simulink model "SigProcess"  (R2022b)
settings: Solver=FixedStepDiscrete  StartTime=0.0  StopTime=10.0  FixedStep=0.001  RelTol=1e-3
undefined symbols (not defined in the file): cClCddAdc_D_u16ADNum, cClCddAdc_D_u8FilterType, cClCddAdc_D_u8RawValueNum, cTmAfCtrl_Te_s32ShttrPosnColdOnHp
libraries: simulink x132
(part 4 of 7)

== system SigProcess/SigProcessSub/Stp4_createSubModInfo/CLHB02001_AdFilter/AVG6 ==
  sigin : Inport
  Compare To Constant : simulink/Logic and Bit Operations/Compare To Constant  relop===  const=0  OutDataTypeStr=boolean
  Constant : Constant  Value=cClCddAdc_D_u8FilterType  OutDataTypeStr=uint8
  Constant1 : Constant  Value=cClCddAdc_D_u8RawValueNum  OutDataTypeStr=uint8
  Counter Limited : simulink/Sources/Counter Limited  uplimit=cClCddAdc_D_u8RawValueNum-1  tsamp=-1
  Data Store Memory : DataStoreMemory  DataStoreName=TempFlapFroLiFbRaw  ReadBeforeWriteMsg=warning  WriteAfterWriteMsg=warning  WriteAfterReadMsg=warning  ShowAdditionalParam=off  OutDataTypeStr=single  Dimensions=[1 20]
      settings: CopyFcn=set_param(gcbh,'ShowName','off');
  Data Store Read : DataStoreRead  DataStoreName=TempFlapFroLiFbRaw  IndexOptions=Index vector (dialog)  Indices=1  OutputSizes=1
  Data Store Write : DataStoreWrite  DataStoreName=TempFlapFroLiFbRaw  DataStoreElements=TempFlapFroLiFbRaw  EnableIndexing=on  IndexMode=Zero-based  IndexOptions=Index vector (port)  Indices=1  OutputSizes=1
  Data Type Conversion : DataTypeConversion  OutDataTypeStr=single  SaturateOnIntegerOverflow=off  RndMeth=Floor
  Gain1 : Gain  Gain=1/cClCddAdc_D_u8RawValueNum
  MATLAB Function : MATLAB Function  TreatAsAtomicUnit=on
  Multiport Switch : MultiPortSwitch  DataPortOrder=Zero-based contiguous  Inputs=5  DataPortForDefault=Additional data port  zeroidx=on  OutDataTypeStr=single  SaturateOnIntegerOverflow=off  InputSameDT=off
  Scope : Scope
  Sum of Elements1 : Sum  Inputs=+
  Switch : Switch  Criteria=u2 ~= 0  SaturateOnIntegerOverflow=off  InputSameDT=off
  Unit Delay : UnitDelay  SampleTime=-1  HasFrameUpgradeWarning=on
  sigAvg : Outport  OutDataTypeStr=single
  wires:
  Data Store Read/1 -> MATLAB Function/1(u), Sum of Elements1/1
  Sum of Elements1/1 -> Gain1/1
  Compare To Constant/1 -> Switch/2
  Switch/1 -> [sigAvgSimple], Unit Delay/1
  Gain1/1 -> Switch/1, [sigAvgQuick]
  Counter Limited/1 -> Compare To Constant/1, Data Store Write/2
  Data Type Conversion/1 -> [siginSingle], Data Store Write/1, Scope/1
  MATLAB Function/2(withoutEdge) -> [sigAvgSortWithoutEdge]
  Unit Delay/1 -> Switch/3
  MATLAB Function/1(mid) -> [sigAvgSortedMid]
  sigin/1 -> [sigin]
  [sigin] -> Data Type Conversion/1
  [sigin] -> Multiport Switch/7
  Constant/1 -> Multiport Switch/1
  [sigAvgSortedMid] -> Multiport Switch/3
  [sigAvgSortWithoutEdge] -> Multiport Switch/4
  [sigAvgSimple] -> Multiport Switch/5
  [sigAvgQuick] -> Multiport Switch/6
  [siginSingle] -> Multiport Switch/2
  Multiport Switch/1 -> [sigAvg]
  [sigAvg] -> sigAvg/1
  Constant1/1 -> MATLAB Function/2(num)

== system SigProcess/SigProcessSub/Stp4_createSubModInfo/CLHB02001_AdFilter/AVG7 ==
  sigin : Inport
  Compare To Constant : simulink/Logic and Bit Operations/Compare To Constant  relop===  const=0  OutDataTypeStr=boolean
  Constant : Constant  Value=cClCddAdc_D_u8FilterType  OutDataTypeStr=uint8
  Constant1 : Constant  Value=cClCddAdc_D_u8RawValueNum  OutDataTypeStr=uint8
  Counter Limited : simulink/Sources/Counter Limited  uplimit=cClCddAdc_D_u8RawValueNum-1  tsamp=-1
  Data Store Memory : DataStoreMemory  DataStoreName=TempFlapFroRIFbRaw  ReadBeforeWriteMsg=warning  WriteAfterWriteMsg=warning  WriteAfterReadMsg=warning  ShowAdditionalParam=off  OutDataTypeStr=single  Dimensions=[1 20]
      settings: CopyFcn=set_param(gcbh,'ShowName','off');
  Data Store Read : DataStoreRead  DataStoreName=TempFlapFroRIFbRaw  IndexOptions=Index vector (dialog)  Indices=1  OutputSizes=1
  Data Store Write : DataStoreWrite  DataStoreName=TempFlapFroRIFbRaw  DataStoreElements=TempFlapFroRIFbRaw  EnableIndexing=on  IndexMode=Zero-based  IndexOptions=Index vector (port)  Indices=1  OutputSizes=1
  Data Type Conversion : DataTypeConversion  OutDataTypeStr=single  SaturateOnIntegerOverflow=off  RndMeth=Floor
  Gain1 : Gain  Gain=1/cClCddAdc_D_u8RawValueNum
  MATLAB Function : MATLAB Function  TreatAsAtomicUnit=on
  Multiport Switch : MultiPortSwitch  DataPortOrder=Zero-based contiguous  Inputs=5  DataPortForDefault=Additional data port  zeroidx=on  OutDataTypeStr=single  SaturateOnIntegerOverflow=off  InputSameDT=off
  Scope : Scope
  Sum of Elements1 : Sum  Inputs=+
  Switch : Switch  Criteria=u2 ~= 0  SaturateOnIntegerOverflow=off  InputSameDT=off
  Unit Delay : UnitDelay  SampleTime=-1  HasFrameUpgradeWarning=on
  sigAvg : Outport  OutDataTypeStr=single
  wires:
  Constant1/1 -> MATLAB Function/2(num)
  [sigAvg] -> sigAvg/1
  Multiport Switch/1 -> [sigAvg]
  [siginSingle] -> Multiport Switch/2
  [sigAvgQuick] -> Multiport Switch/6
  [sigAvgSimple] -> Multiport Switch/5
  [sigAvgSortWithoutEdge] -> Multiport Switch/4
  [sigAvgSortedMid] -> Multiport Switch/3
  Constant/1 -> Multiport Switch/1
  [sigin] -> Multiport Switch/7
  [sigin] -> Data Type Conversion/1
  sigin/1 -> [sigin]
  MATLAB Function/1(mid) -> [sigAvgSortedMid]
  Unit Delay/1 -> Switch/3
  MATLAB Function/2(withoutEdge) -> [sigAvgSortWithoutEdge]
  Data Type Conversion/1 -> Scope/1, Data Store Write/1, [siginSingle]
  Counter Limited/1 -> Data Store Write/2, Compare To Constant/1
  Gain1/1 -> [sigAvgQuick], Switch/1
  Switch/1 -> Unit Delay/1, [sigAvgSimple]
  Compare To Constant/1 -> Switch/2
  Sum of Elements1/1 -> Gain1/1
  Data Store Read/1 -> Sum of Elements1/1, MATLAB Function/1(u)

== system SigProcess/SigProcessSub/Stp4_createSubModInfo/CLHB02001_AdFilter/AVG8 ==
  sigin : Inport
  Compare To Constant : simulink/Logic and Bit Operations/Compare To Constant  relop===  const=0  OutDataTypeStr=boolean
  Constant : Constant  Value=cClCddAdc_D_u8FilterType  OutDataTypeStr=uint8
  Constant1 : Constant  Value=cClCddAdc_D_u8RawValueNum  OutDataTypeStr=uint8
  Counter Limited : simulink/Sources/Counter Limited  uplimit=cClCddAdc_D_u8RawValueNum-1  tsamp=-1
  Data Store Memory : DataStoreMemory  DataStoreName=ModFlapFroRIFbRaw  ReadBeforeWriteMsg=warning  WriteAfterWriteMsg=warning  WriteAfterReadMsg=warning  ShowAdditionalParam=off  OutDataTypeStr=single  Dimensions=[1 20]
      settings: CopyFcn=set_param(gcbh,'ShowName','off');
  Data Store Read : DataStoreRead  DataStoreName=ModFlapFroRIFbRaw  IndexOptions=Index vector (dialog)  Indices=1  OutputSizes=1
  Data Store Write : DataStoreWrite  DataStoreName=ModFlapFroRIFbRaw  DataStoreElements=ModFlapFroRIFbRaw  EnableIndexing=on  IndexMode=Zero-based  IndexOptions=Index vector (port)  Indices=1  OutputSizes=1
  Data Type Conversion : DataTypeConversion  OutDataTypeStr=single  SaturateOnIntegerOverflow=off  RndMeth=Floor
  Gain1 : Gain  Gain=1/cClCddAdc_D_u8RawValueNum
  MATLAB Function : MATLAB Function  TreatAsAtomicUnit=on
  Multiport Switch : MultiPortSwitch  DataPortOrder=Zero-based contiguous  Inputs=5  DataPortForDefault=Additional data port  zeroidx=on  OutDataTypeStr=single  SaturateOnIntegerOverflow=off  InputSameDT=off
  Scope : Scope
  Sum of Elements1 : Sum  Inputs=+
  Switch : Switch  Criteria=u2 ~= 0  SaturateOnIntegerOverflow=off  InputSameDT=off
  Unit Delay : UnitDelay  SampleTime=-1  HasFrameUpgradeWarning=on
  sigAvg : Outport  OutDataTypeStr=single
  wires:
  Data Store Read/1 -> MATLAB Function/1(u), Sum of Elements1/1
  Sum of Elements1/1 -> Gain1/1
  Compare To Constant/1 -> Switch/2
  Switch/1 -> [sigAvgSimple], Unit Delay/1
  Gain1/1 -> Switch/1, [sigAvgQuick]
  Counter Limited/1 -> Compare To Constant/1, Data Store Write/2
  Data Type Conversion/1 -> [siginSingle], Data Store Write/1, Scope/1
  MATLAB Function/2(withoutEdge) -> [sigAvgSortWithoutEdge]
  Unit Delay/1 -> Switch/3
  MATLAB Function/1(mid) -> [sigAvgSortedMid]
  sigin/1 -> [sigin]
  [sigin] -> Data Type Conversion/1
  [sigin] -> Multiport Switch/7
  Constant/1 -> Multiport Switch/1
  [sigAvgSortedMid] -> Multiport Switch/3
  [sigAvgSortWithoutEdge] -> Multiport Switch/4
  [sigAvgSimple] -> Multiport Switch/5
  [sigAvgQuick] -> Multiport Switch/6
  [siginSingle] -> Multiport Switch/2
  Multiport Switch/1 -> [sigAvg]
  [sigAvg] -> sigAvg/1
  Constant1/1 -> MATLAB Function/2(num)

== system SigProcess/SigProcessSub/Stp4_createSubModInfo/CLHB02001_AdFilter/AVG9 ==
  sigin : Inport
  Compare To Constant : simulink/Logic and Bit Operations/Compare To Constant  relop===  const=0  OutDataTypeStr=boolean
  Constant : Constant  Value=cClCddAdc_D_u8FilterType  OutDataTypeStr=uint8
  Constant1 : Constant  Value=cClCddAdc_D_u8RawValueNum  OutDataTypeStr=uint8
  Counter Limited : simulink/Sources/Counter Limited  uplimit=cClCddAdc_D_u8RawValueNum-1  tsamp=-1
  Data Store Memory : DataStoreMemory  DataStoreName=AqsPinRaw  ReadBeforeWriteMsg=warning  WriteAfterWriteMsg=warning  WriteAfterReadMsg=warning  ShowAdditionalParam=off  OutDataTypeStr=single  Dimensions=[1 20]
      settings: CopyFcn=set_param(gcbh,'ShowName','off');
  Data Store Read : DataStoreRead  DataStoreName=AqsPinRaw  IndexOptions=Index vector (dialog)  Indices=1  OutputSizes=1
  Data Store Write : DataStoreWrite  DataStoreName=AqsPinRaw  DataStoreElements=AqsPinRaw  EnableIndexing=on  IndexMode=Zero-based  IndexOptions=Index vector (port)  Indices=1  OutputSizes=1
  Data Type Conversion : DataTypeConversion  OutDataTypeStr=single  SaturateOnIntegerOverflow=off  RndMeth=Floor
  Gain1 : Gain  Gain=1/cClCddAdc_D_u8RawValueNum
  MATLAB Function : MATLAB Function  TreatAsAtomicUnit=on
  Multiport Switch : MultiPortSwitch  DataPortOrder=Zero-based contiguous  Inputs=5  DataPortForDefault=Additional data port  zeroidx=on  OutDataTypeStr=single  SaturateOnIntegerOverflow=off  InputSameDT=off
  Scope : Scope
  Sum of Elements1 : Sum  Inputs=+
  Switch : Switch  Criteria=u2 ~= 0  SaturateOnIntegerOverflow=off  InputSameDT=off
  Unit Delay : UnitDelay  SampleTime=-1  HasFrameUpgradeWarning=on
  sigAvg : Outport  OutDataTypeStr=single
  wires:
  Constant1/1 -> MATLAB Function/2(num)
  [sigAvg] -> sigAvg/1
  Multiport Switch/1 -> [sigAvg]
  [siginSingle] -> Multiport Switch/2
  [sigAvgQuick] -> Multiport Switch/6
  [sigAvgSimple] -> Multiport Switch/5
  [sigAvgSortWithoutEdge] -> Multiport Switch/4
  [sigAvgSortedMid] -> Multiport Switch/3
  Constant/1 -> Multiport Switch/1
  [sigin] -> Multiport Switch/7
  [sigin] -> Data Type Conversion/1
  sigin/1 -> [sigin]
  MATLAB Function/1(mid) -> [sigAvgSortedMid]
  Unit Delay/1 -> Switch/3
  MATLAB Function/2(withoutEdge) -> [sigAvgSortWithoutEdge]
  Data Type Conversion/1 -> Scope/1, Data Store Write/1, [siginSingle]
  Counter Limited/1 -> Data Store Write/2, Compare To Constant/1
  Gain1/1 -> [sigAvgQuick], Switch/1
  Switch/1 -> Unit Delay/1, [sigAvgSimple]
  Compare To Constant/1 -> Switch/2
  Sum of Elements1/1 -> Gain1/1
  Data Store Read/1 -> Sum of Elements1/1, MATLAB Function/1(u)

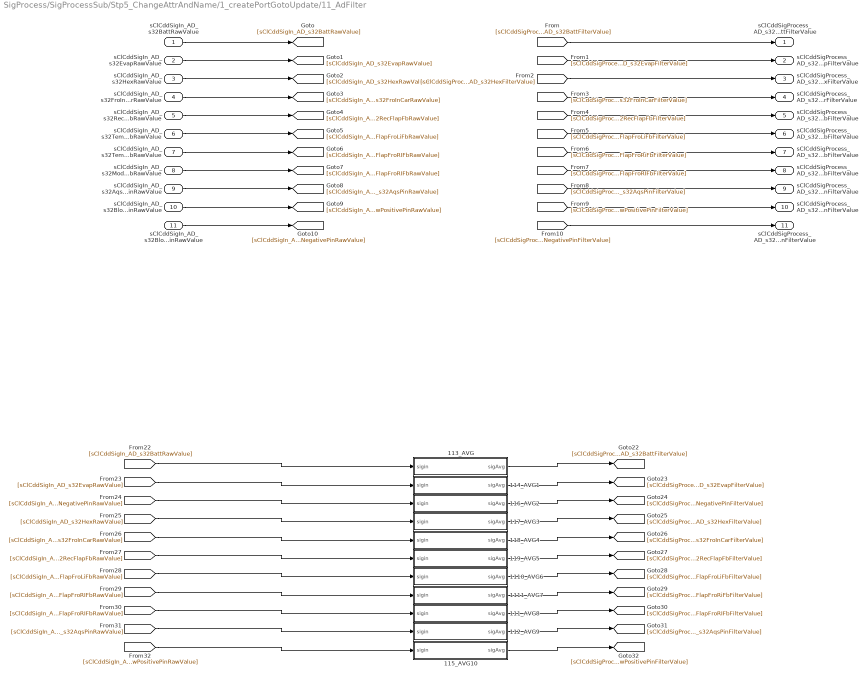
== system SigProcess/SigProcessSub/Stp5_ChangeAttrAndName/1_createPortGotoUpdate/11_AdFilter ==
  sClCddSigIn_AD_s32BattRawValue : Inport  Description=低压电池AD值  OutDataTypeStr=single
  sClCddSigIn_AD_s32EvapRawValue : Inport  Description=空调箱蒸发器原始AD值  Port=2  OutDataTypeStr=single
  sClCddSigIn_AD_s32HexRawValue : Inport  Description=空调箱热交换器原始AD值  Port=3  OutDataTypeStr=single
  sClCddSigIn_AD_s32FroInCarRawValue : Inport  Description=前排车内温度传感器AD值  Port=4  OutDataTypeStr=single
  sClCddSigIn_AD_s32RecFlapFbRawValue : Inport  Description=内循环风门电机位置反馈  Port=5  OutDataTypeStr=single
  sClCddSigIn_AD_s32TempFlapFroLiFbRawValue : Inport  Description=前左风门电机位置反馈  Port=6  OutDataTypeStr=single
  sClCddSigIn_AD_s32TempFlapFroRIFbRawValue : Inport  Description=前右风门电机位置反馈  Port=7  OutMin=0  OutMax=2048  OutDataTypeStr=single
  sClCddSigIn_AD_s32ModFlapFroRIFbRawValue : Inport  Description=模式风门电机位置反馈  Port=8  OutMin=0  OutMax=2048  OutDataTypeStr=single
  sClCddSigIn_AD_s32AqsPinRawValue : Inport  Description=AQSPWM驱动芯片诊断PIN脚AD值  Port=9  OutMin=0  OutMax=2048  OutDataTypeStr=single
  sClCddSigIn_AD_s32BlowPositivePinRawValue : Inport  Description=鼓风机调速电机正极反馈  Port=10  OutMin=0  OutMax=2048  OutDataTypeStr=single
  sClCddSigIn_AD_s32BlowNegativePinRawValue : Inport  Description=鼓风机调速电机负极反馈  Port=11  OutMin=0  OutMax=2048  OutDataTypeStr=single
  1110_AVG6 : Subsystem
  1111_AVG7 : Subsystem
  111_AVG8 : Subsystem
  112_AVG9 : Subsystem
  113_AVG : Subsystem
  114_AVG1 : Subsystem
  115_AVG10 : Subsystem
  116_AVG2 : Subsystem
  117_AVG3 : Subsystem
  118_AVG4 : Subsystem
  119_AVG5 : Subsystem
  sClCddSigProcess_AD_s32BattFilterValue : Outport  Description=低压电池滤波后AD值  OutMin=0  OutMax=2048  OutDataTypeStr=single
  sClCddSigProcess_AD_s32EvapFilterValue : Outport  Description=空调箱蒸发器滤波后AD值  Port=2  OutMin=0  OutMax=2048  OutDataTypeStr=single
  sClCddSigProcess_AD_s32HexFilterValue : Outport  Description=空调箱热交换器滤波后AD值  Port=3  OutMin=0  OutMax=2048  OutDataTypeStr=single
  sClCddSigProcess_AD_s32FroInCarFilterValue : Outport  Description=前排车内温度传感器滤波后AD值  Port=4  OutMin=0  OutMax=2048  OutDataTypeStr=single
  sClCddSigProcess_AD_s32RecFlapFbFilterValue : Outport  Description=内循环风门电机位置反馈滤波值  Port=5  OutMin=0  OutMax=2048  OutDataTypeStr=single
  sClCddSigProcess_AD_s32TempFlapFroLiFbFilterValue : Outport  Description=前左风门电机位置反馈滤波值  Port=6  OutMin=0  OutMax=2048  OutDataTypeStr=single
  sClCddSigProcess_AD_s32TempFlapFroRiFbFilterValue : Outport  Description=前右风门电机位置反馈滤波值  Port=7  OutMin=0  OutMax=2048  OutDataTypeStr=single
  sClCddSigProcess_AD_s32ModFlapFroRIFbFilterValue : Outport  Description=模式风门电机位置反馈滤波值  Port=8  OutMin=0  OutMax=2048  OutDataTypeStr=single
  sClCddSigProcess_AD_s32AqsPinFilterValue : Outport  Description=AQSPWM驱动芯片诊断PIN脚滤波值  Port=9  OutMin=0  OutMax=2048  OutDataTypeStr=single
  sClCddSigProcess_AD_s32BlowPositivePinFilterValue : Outport  Description=鼓风机调速电机正极反馈滤波值  Port=10  OutMin=0  OutMax=2048  OutDataTypeStr=single
  sClCddSigProcess_AD_s32BlowNegativePinFilterValue : Outport  Description=鼓风机调速电机负极反馈滤波值  Port=11  OutMin=0  OutMax=2048  OutDataTypeStr=single
  wires:
  [sClCddSigProcess_AD_s32BlowNegativePinFilterValue] -> sClCddSigProcess_AD_s32BlowNegativePinFilterValue/1
  [sClCddSigProcess_AD_s32BlowPositivePinFilterValue] -> sClCddSigProcess_AD_s32BlowPositivePinFilterValue/1
  [sClCddSigProcess_AD_s32AqsPinFilterValue] -> sClCddSigProcess_AD_s32AqsPinFilterValue/1
  [sClCddSigProcess_AD_s32ModFlapFroRIFbFilterValue] -> sClCddSigProcess_AD_s32ModFlapFroRIFbFilterValue/1
  [sClCddSigProcess_AD_s32TempFlapFroRiFbFilterValue] -> sClCddSigProcess_AD_s32TempFlapFroRiFbFilterValue/1
  [sClCddSigProcess_AD_s32TempFlapFroLiFbFilterValue] -> sClCddSigProcess_AD_s32TempFlapFroLiFbFilterValue/1
  [sClCddSigProcess_AD_s32RecFlapFbFilterValue] -> sClCddSigProcess_AD_s32RecFlapFbFilterValue/1
  [sClCddSigProcess_AD_s32FroInCarFilterValue] -> sClCddSigProcess_AD_s32FroInCarFilterValue/1
  [sClCddSigProcess_AD_s32HexFilterValue] -> sClCddSigProcess_AD_s32HexFilterValue/1
  [sClCddSigProcess_AD_s32EvapFilterValue] -> sClCddSigProcess_AD_s32EvapFilterValue/1
  [sClCddSigProcess_AD_s32BattFilterValue] -> sClCddSigProcess_AD_s32BattFilterValue/1
  sClCddSigIn_AD_s32BlowNegativePinRawValue/1 -> [sClCddSigIn_AD_s32BlowNegativePinRawValue]
  sClCddSigIn_AD_s32BlowPositivePinRawValue/1 -> [sClCddSigIn_AD_s32BlowPositivePinRawValue]
  sClCddSigIn_AD_s32AqsPinRawValue/1 -> [sClCddSigIn_AD_s32AqsPinRawValue]
  sClCddSigIn_AD_s32ModFlapFroRIFbRawValue/1 -> [sClCddSigIn_AD_s32ModFlapFroRIFbRawValue]
  sClCddSigIn_AD_s32TempFlapFroRIFbRawValue/1 -> [sClCddSigIn_AD_s32TempFlapFroRIFbRawValue]
  sClCddSigIn_AD_s32TempFlapFroLiFbRawValue/1 -> [sClCddSigIn_AD_s32TempFlapFroLiFbRawValue]
  sClCddSigIn_AD_s32RecFlapFbRawValue/1 -> [sClCddSigIn_AD_s32RecFlapFbRawValue]
  sClCddSigIn_AD_s32FroInCarRawValue/1 -> [sClCddSigIn_AD_s32FroInCarRawValue]
  sClCddSigIn_AD_s32HexRawValue/1 -> [sClCddSigIn_AD_s32HexRawValue]
  sClCddSigIn_AD_s32EvapRawValue/1 -> [sClCddSigIn_AD_s32EvapRawValue]
  sClCddSigIn_AD_s32BattRawValue/1 -> [sClCddSigIn_AD_s32BattRawValue]
  [sClCddSigIn_AD_s32RecFlapFbRawValue] -> 119_AVG5/1(sigin)
  111_AVG8/1(sigAvg) -> [sClCddSigProcess_AD_s32ModFlapFroRIFbFilterValue]
  115_AVG10/1(sigAvg) -> [sClCddSigProcess_AD_s32BlowPositivePinFilterValue]
  [sClCddSigIn_AD_s32AqsPinRawValue] -> 112_AVG9/1(sigin)
  112_AVG9/1(sigAvg) -> [sClCddSigProcess_AD_s32AqsPinFilterValue]
  1110_AVG6/1(sigAvg) -> [sClCddSigProcess_AD_s32TempFlapFroLiFbFilterValue]
  [sClCddSigIn_AD_s32ModFlapFroRIFbRawValue] -> 111_AVG8/1(sigin)
  [sClCddSigIn_AD_s32BlowNegativePinRawValue] -> 116_AVG2/1(sigin)
  [sClCddSigIn_AD_s32EvapRawValue] -> 114_AVG1/1(sigin)
  [sClCddSigIn_AD_s32BattRawValue] -> 113_AVG/1(sigin)
  113_AVG/1(sigAvg) -> [sClCddSigProcess_AD_s32BattFilterValue]
  114_AVG1/1(sigAvg) -> [sClCddSigProcess_AD_s32EvapFilterValue]
  119_AVG5/1(sigAvg) -> [sClCddSigProcess_AD_s32RecFlapFbFilterValue]
  [sClCddSigIn_AD_s32FroInCarRawValue] -> 118_AVG4/1(sigin)
  118_AVG4/1(sigAvg) -> [sClCddSigProcess_AD_s32FroInCarFilterValue]
  116_AVG2/1(sigAvg) -> [sClCddSigProcess_AD_s32BlowNegativePinFilterValue]
  [sClCddSigIn_AD_s32TempFlapFroRIFbRawValue] -> 1111_AVG7/1(sigin)
  [sClCddSigIn_AD_s32BlowPositivePinRawValue] -> 115_AVG10/1(sigin)
  [sClCddSigIn_AD_s32HexRawValue] -> 117_AVG3/1(sigin)
  117_AVG3/1(sigAvg) -> [sClCddSigProcess_AD_s32HexFilterValue]
  [sClCddSigIn_AD_s32TempFlapFroLiFbRawValue] -> 1110_AVG6/1(sigin)
  1111_AVG7/1(sigAvg) -> [sClCddSigProcess_AD_s32TempFlapFroRiFbFilterValue]

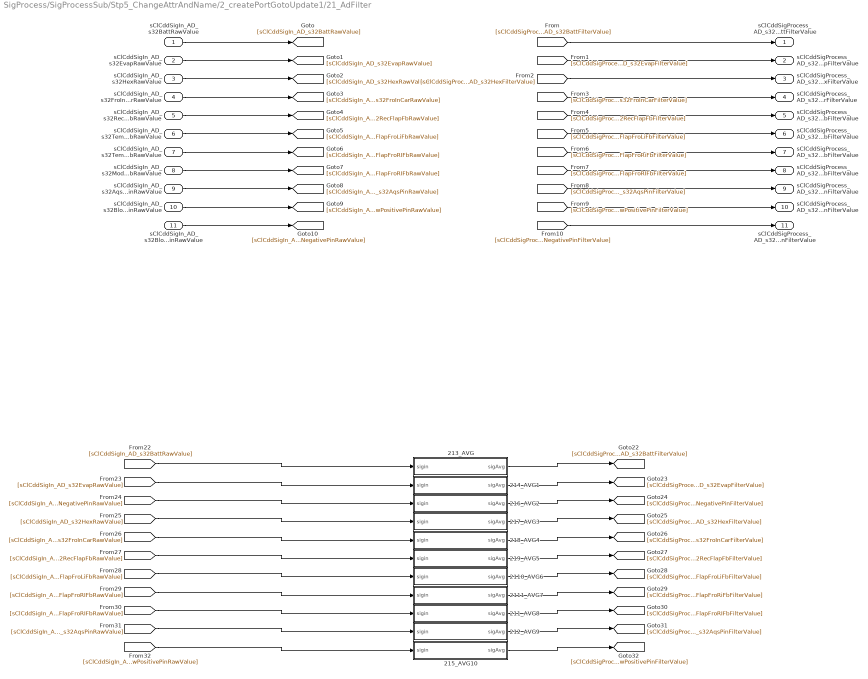
== system SigProcess/SigProcessSub/Stp5_ChangeAttrAndName/2_createPortGotoUpdate1/21_AdFilter ==
  sClCddSigIn_AD_s32BattRawValue : Inport  Description=低压电池AD值  OutDataTypeStr=single
  sClCddSigIn_AD_s32EvapRawValue : Inport  Description=空调箱蒸发器原始AD值  Port=2  OutDataTypeStr=single
  sClCddSigIn_AD_s32HexRawValue : Inport  Description=空调箱热交换器原始AD值  Port=3  OutDataTypeStr=single
  sClCddSigIn_AD_s32FroInCarRawValue : Inport  Description=前排车内温度传感器AD值  Port=4  OutDataTypeStr=single
  sClCddSigIn_AD_s32RecFlapFbRawValue : Inport  Description=内循环风门电机位置反馈  Port=5  OutDataTypeStr=single
  sClCddSigIn_AD_s32TempFlapFroLiFbRawValue : Inport  Description=前左风门电机位置反馈  Port=6  OutDataTypeStr=single
  sClCddSigIn_AD_s32TempFlapFroRIFbRawValue : Inport  Description=前右风门电机位置反馈  Port=7  OutMin=0  OutMax=2048  OutDataTypeStr=single
  sClCddSigIn_AD_s32ModFlapFroRIFbRawValue : Inport  Description=模式风门电机位置反馈  Port=8  OutMin=0  OutMax=2048  OutDataTypeStr=single
  sClCddSigIn_AD_s32AqsPinRawValue : Inport  Description=AQSPWM驱动芯片诊断PIN脚AD值  Port=9  OutMin=0  OutMax=2048  OutDataTypeStr=single
  sClCddSigIn_AD_s32BlowPositivePinRawValue : Inport  Description=鼓风机调速电机正极反馈  Port=10  OutMin=0  OutMax=2048  OutDataTypeStr=single
  sClCddSigIn_AD_s32BlowNegativePinRawValue : Inport  Description=鼓风机调速电机负极反馈  Port=11  OutMin=0  OutMax=2048  OutDataTypeStr=single
  2110_AVG6 : Subsystem
  2111_AVG7 : Subsystem
  211_AVG8 : Subsystem
  212_AVG9 : Subsystem
  213_AVG : Subsystem
  214_AVG1 : Subsystem
  215_AVG10 : Subsystem
  216_AVG2 : Subsystem
  217_AVG3 : Subsystem
  218_AVG4 : Subsystem
  219_AVG5 : Subsystem
  sClCddSigProcess_AD_s32BattFilterValue : Outport  Description=低压电池滤波后AD值  OutMin=0  OutMax=2048  OutDataTypeStr=single
  sClCddSigProcess_AD_s32EvapFilterValue : Outport  Description=空调箱蒸发器滤波后AD值  Port=2  OutMin=0  OutMax=2048  OutDataTypeStr=single
  sClCddSigProcess_AD_s32HexFilterValue : Outport  Description=空调箱热交换器滤波后AD值  Port=3  OutMin=0  OutMax=2048  OutDataTypeStr=single
  sClCddSigProcess_AD_s32FroInCarFilterValue : Outport  Description=前排车内温度传感器滤波后AD值  Port=4  OutMin=0  OutMax=2048  OutDataTypeStr=single
  sClCddSigProcess_AD_s32RecFlapFbFilterValue : Outport  Description=内循环风门电机位置反馈滤波值  Port=5  OutMin=0  OutMax=2048  OutDataTypeStr=single
  sClCddSigProcess_AD_s32TempFlapFroLiFbFilterValue : Outport  Description=前左风门电机位置反馈滤波值  Port=6  OutMin=0  OutMax=2048  OutDataTypeStr=single
  sClCddSigProcess_AD_s32TempFlapFroRiFbFilterValue : Outport  Description=前右风门电机位置反馈滤波值  Port=7  OutMin=0  OutMax=2048  OutDataTypeStr=single
  sClCddSigProcess_AD_s32ModFlapFroRIFbFilterValue : Outport  Description=模式风门电机位置反馈滤波值  Port=8  OutMin=0  OutMax=2048  OutDataTypeStr=single
  sClCddSigProcess_AD_s32AqsPinFilterValue : Outport  Description=AQSPWM驱动芯片诊断PIN脚滤波值  Port=9  OutMin=0  OutMax=2048  OutDataTypeStr=single
  sClCddSigProcess_AD_s32BlowPositivePinFilterValue : Outport  Description=鼓风机调速电机正极反馈滤波值  Port=10  OutMin=0  OutMax=2048  OutDataTypeStr=single
  sClCddSigProcess_AD_s32BlowNegativePinFilterValue : Outport  Description=鼓风机调速电机负极反馈滤波值  Port=11  OutMin=0  OutMax=2048  OutDataTypeStr=single
  wires:
  2111_AVG7/1(sigAvg) -> [sClCddSigProcess_AD_s32TempFlapFroRiFbFilterValue]
  [sClCddSigIn_AD_s32TempFlapFroLiFbRawValue] -> 2110_AVG6/1(sigin)
  217_AVG3/1(sigAvg) -> [sClCddSigProcess_AD_s32HexFilterValue]
  [sClCddSigIn_AD_s32HexRawValue] -> 217_AVG3/1(sigin)
  [sClCddSigIn_AD_s32BlowPositivePinRawValue] -> 215_AVG10/1(sigin)
  [sClCddSigIn_AD_s32TempFlapFroRIFbRawValue] -> 2111_AVG7/1(sigin)
  216_AVG2/1(sigAvg) -> [sClCddSigProcess_AD_s32BlowNegativePinFilterValue]
  218_AVG4/1(sigAvg) -> [sClCddSigProcess_AD_s32FroInCarFilterValue]
  [sClCddSigIn_AD_s32FroInCarRawValue] -> 218_AVG4/1(sigin)
  219_AVG5/1(sigAvg) -> [sClCddSigProcess_AD_s32RecFlapFbFilterValue]
  214_AVG1/1(sigAvg) -> [sClCddSigProcess_AD_s32EvapFilterValue]
  213_AVG/1(sigAvg) -> [sClCddSigProcess_AD_s32BattFilterValue]
  [sClCddSigIn_AD_s32BattRawValue] -> 213_AVG/1(sigin)
  [sClCddSigIn_AD_s32EvapRawValue] -> 214_AVG1/1(sigin)
  [sClCddSigIn_AD_s32BlowNegativePinRawValue] -> 216_AVG2/1(sigin)
  [sClCddSigIn_AD_s32ModFlapFroRIFbRawValue] -> 211_AVG8/1(sigin)
  2110_AVG6/1(sigAvg) -> [sClCddSigProcess_AD_s32TempFlapFroLiFbFilterValue]
  212_AVG9/1(sigAvg) -> [sClCddSigProcess_AD_s32AqsPinFilterValue]
  [sClCddSigIn_AD_s32AqsPinRawValue] -> 212_AVG9/1(sigin)
  215_AVG10/1(sigAvg) -> [sClCddSigProcess_AD_s32BlowPositivePinFilterValue]
  211_AVG8/1(sigAvg) -> [sClCddSigProcess_AD_s32ModFlapFroRIFbFilterValue]
  [sClCddSigIn_AD_s32RecFlapFbRawValue] -> 219_AVG5/1(sigin)
  sClCddSigIn_AD_s32BattRawValue/1 -> [sClCddSigIn_AD_s32BattRawValue]
  sClCddSigIn_AD_s32EvapRawValue/1 -> [sClCddSigIn_AD_s32EvapRawValue]
  sClCddSigIn_AD_s32HexRawValue/1 -> [sClCddSigIn_AD_s32HexRawValue]
  sClCddSigIn_AD_s32FroInCarRawValue/1 -> [sClCddSigIn_AD_s32FroInCarRawValue]
  sClCddSigIn_AD_s32RecFlapFbRawValue/1 -> [sClCddSigIn_AD_s32RecFlapFbRawValue]
  sClCddSigIn_AD_s32TempFlapFroLiFbRawValue/1 -> [sClCddSigIn_AD_s32TempFlapFroLiFbRawValue]
  sClCddSigIn_AD_s32TempFlapFroRIFbRawValue/1 -> [sClCddSigIn_AD_s32TempFlapFroRIFbRawValue]
  sClCddSigIn_AD_s32ModFlapFroRIFbRawValue/1 -> [sClCddSigIn_AD_s32ModFlapFroRIFbRawValue]
  sClCddSigIn_AD_s32AqsPinRawValue/1 -> [sClCddSigIn_AD_s32AqsPinRawValue]
  sClCddSigIn_AD_s32BlowPositivePinRawValue/1 -> [sClCddSigIn_AD_s32BlowPositivePinRawValue]
  sClCddSigIn_AD_s32BlowNegativePinRawValue/1 -> [sClCddSigIn_AD_s32BlowNegativePinRawValue]
  [sClCddSigProcess_AD_s32BattFilterValue] -> sClCddSigProcess_AD_s32BattFilterValue/1
  [sClCddSigProcess_AD_s32EvapFilterValue] -> sClCddSigProcess_AD_s32EvapFilterValue/1
  [sClCddSigProcess_AD_s32HexFilterValue] -> sClCddSigProcess_AD_s32HexFilterValue/1
  [sClCddSigProcess_AD_s32FroInCarFilterValue] -> sClCddSigProcess_AD_s32FroInCarFilterValue/1
  [sClCddSigProcess_AD_s32RecFlapFbFilterValue] -> sClCddSigProcess_AD_s32RecFlapFbFilterValue/1
  [sClCddSigProcess_AD_s32TempFlapFroLiFbFilterValue] -> sClCddSigProcess_AD_s32TempFlapFroLiFbFilterValue/1
  [sClCddSigProcess_AD_s32TempFlapFroRiFbFilterValue] -> sClCddSigProcess_AD_s32TempFlapFroRiFbFilterValue/1
  [sClCddSigProcess_AD_s32ModFlapFroRIFbFilterValue] -> sClCddSigProcess_AD_s32ModFlapFroRIFbFilterValue/1
  [sClCddSigProcess_AD_s32AqsPinFilterValue] -> sClCddSigProcess_AD_s32AqsPinFilterValue/1
  [sClCddSigProcess_AD_s32BlowPositivePinFilterValue] -> sClCddSigProcess_AD_s32BlowPositivePinFilterValue/1
  [sClCddSigProcess_AD_s32BlowNegativePinFilterValue] -> sClCddSigProcess_AD_s32BlowNegativePinFilterValue/1

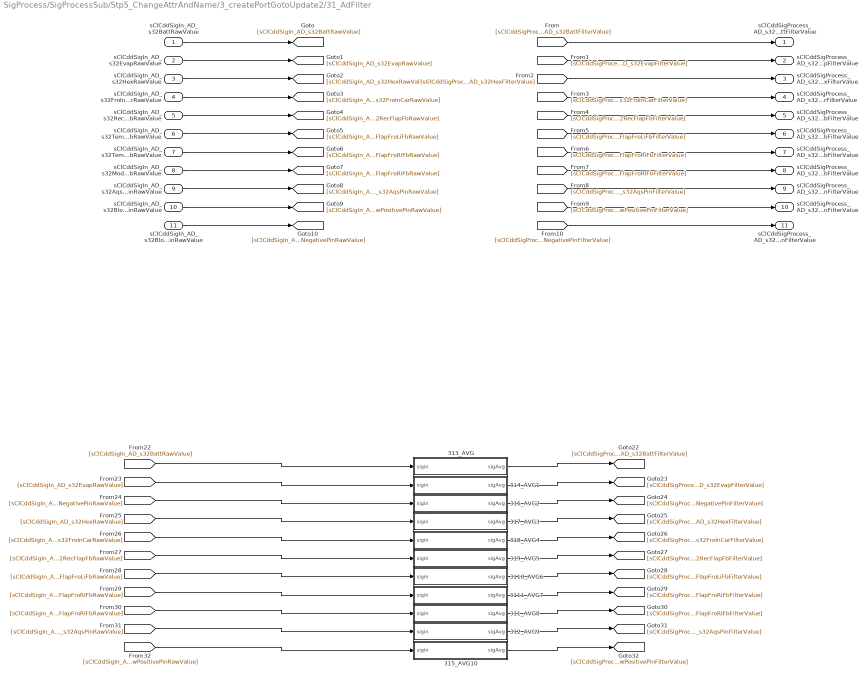
== system SigProcess/SigProcessSub/Stp5_ChangeAttrAndName/3_createPortGotoUpdate2/31_AdFilter ==
  sClCddSigIn_AD_s32BattRawValue : Inport  Description=低压电池AD值  OutDataTypeStr=single
  sClCddSigIn_AD_s32EvapRawValue : Inport  Description=空调箱蒸发器原始AD值  Port=2  OutDataTypeStr=single
  sClCddSigIn_AD_s32HexRawValue : Inport  Description=空调箱热交换器原始AD值  Port=3  OutDataTypeStr=single
  sClCddSigIn_AD_s32FroInCarRawValue : Inport  Description=前排车内温度传感器AD值  Port=4  OutDataTypeStr=single
  sClCddSigIn_AD_s32RecFlapFbRawValue : Inport  Description=内循环风门电机位置反馈  Port=5  OutDataTypeStr=single
  sClCddSigIn_AD_s32TempFlapFroLiFbRawValue : Inport  Description=前左风门电机位置反馈  Port=6  OutDataTypeStr=single
  sClCddSigIn_AD_s32TempFlapFroRIFbRawValue : Inport  Description=前右风门电机位置反馈  Port=7  OutMin=0  OutMax=2048  OutDataTypeStr=single
  sClCddSigIn_AD_s32ModFlapFroRIFbRawValue : Inport  Description=模式风门电机位置反馈  Port=8  OutMin=0  OutMax=2048  OutDataTypeStr=single
  sClCddSigIn_AD_s32AqsPinRawValue : Inport  Description=AQSPWM驱动芯片诊断PIN脚AD值  Port=9  OutMin=0  OutMax=2048  OutDataTypeStr=single
  sClCddSigIn_AD_s32BlowPositivePinRawValue : Inport  Description=鼓风机调速电机正极反馈  Port=10  OutMin=0  OutMax=2048  OutDataTypeStr=single
  sClCddSigIn_AD_s32BlowNegativePinRawValue : Inport  Description=鼓风机调速电机负极反馈  Port=11  OutMin=0  OutMax=2048  OutDataTypeStr=single
  3110_AVG6 : Subsystem
  3111_AVG7 : Subsystem
  311_AVG8 : Subsystem
  312_AVG9 : Subsystem
  313_AVG : Subsystem
  314_AVG1 : Subsystem
  315_AVG10 : Subsystem
  316_AVG2 : Subsystem
  317_AVG3 : Subsystem
  318_AVG4 : Subsystem
  319_AVG5 : Subsystem
  sClCddSigProcess_AD_s32BattFilterValue : Outport  Description=低压电池滤波后AD值  OutMin=0  OutMax=2048  OutDataTypeStr=single
  sClCddSigProcess_AD_s32EvapFilterValue : Outport  Description=空调箱蒸发器滤波后AD值  Port=2  OutMin=0  OutMax=2048  OutDataTypeStr=single
  sClCddSigProcess_AD_s32HexFilterValue : Outport  Description=空调箱热交换器滤波后AD值  Port=3  OutMin=0  OutMax=2048  OutDataTypeStr=single
  sClCddSigProcess_AD_s32FroInCarFilterValue : Outport  Description=前排车内温度传感器滤波后AD值  Port=4  OutMin=0  OutMax=2048  OutDataTypeStr=single
  sClCddSigProcess_AD_s32RecFlapFbFilterValue : Outport  Description=内循环风门电机位置反馈滤波值  Port=5  OutMin=0  OutMax=2048  OutDataTypeStr=single
  sClCddSigProcess_AD_s32TempFlapFroLiFbFilterValue : Outport  Description=前左风门电机位置反馈滤波值  Port=6  OutMin=0  OutMax=2048  OutDataTypeStr=single
  sClCddSigProcess_AD_s32TempFlapFroRiFbFilterValue : Outport  Description=前右风门电机位置反馈滤波值  Port=7  OutMin=0  OutMax=2048  OutDataTypeStr=single
  sClCddSigProcess_AD_s32ModFlapFroRIFbFilterValue : Outport  Description=模式风门电机位置反馈滤波值  Port=8  OutMin=0  OutMax=2048  OutDataTypeStr=single
  sClCddSigProcess_AD_s32AqsPinFilterValue : Outport  Description=AQSPWM驱动芯片诊断PIN脚滤波值  Port=9  OutMin=0  OutMax=2048  OutDataTypeStr=single
  sClCddSigProcess_AD_s32BlowPositivePinFilterValue : Outport  Description=鼓风机调速电机正极反馈滤波值  Port=10  OutMin=0  OutMax=2048  OutDataTypeStr=single
  sClCddSigProcess_AD_s32BlowNegativePinFilterValue : Outport  Description=鼓风机调速电机负极反馈滤波值  Port=11  OutMin=0  OutMax=2048  OutDataTypeStr=single
  wires:
  [sClCddSigProcess_AD_s32BlowNegativePinFilterValue] -> sClCddSigProcess_AD_s32BlowNegativePinFilterValue/1
  [sClCddSigProcess_AD_s32BlowPositivePinFilterValue] -> sClCddSigProcess_AD_s32BlowPositivePinFilterValue/1
  [sClCddSigProcess_AD_s32AqsPinFilterValue] -> sClCddSigProcess_AD_s32AqsPinFilterValue/1
  [sClCddSigProcess_AD_s32ModFlapFroRIFbFilterValue] -> sClCddSigProcess_AD_s32ModFlapFroRIFbFilterValue/1
  [sClCddSigProcess_AD_s32TempFlapFroRiFbFilterValue] -> sClCddSigProcess_AD_s32TempFlapFroRiFbFilterValue/1
  [sClCddSigProcess_AD_s32TempFlapFroLiFbFilterValue] -> sClCddSigProcess_AD_s32TempFlapFroLiFbFilterValue/1
  [sClCddSigProcess_AD_s32RecFlapFbFilterValue] -> sClCddSigProcess_AD_s32RecFlapFbFilterValue/1
  [sClCddSigProcess_AD_s32FroInCarFilterValue] -> sClCddSigProcess_AD_s32FroInCarFilterValue/1
  [sClCddSigProcess_AD_s32HexFilterValue] -> sClCddSigProcess_AD_s32HexFilterValue/1
  [sClCddSigProcess_AD_s32EvapFilterValue] -> sClCddSigProcess_AD_s32EvapFilterValue/1
  [sClCddSigProcess_AD_s32BattFilterValue] -> sClCddSigProcess_AD_s32BattFilterValue/1
  sClCddSigIn_AD_s32BlowNegativePinRawValue/1 -> [sClCddSigIn_AD_s32BlowNegativePinRawValue]
  sClCddSigIn_AD_s32BlowPositivePinRawValue/1 -> [sClCddSigIn_AD_s32BlowPositivePinRawValue]
  sClCddSigIn_AD_s32AqsPinRawValue/1 -> [sClCddSigIn_AD_s32AqsPinRawValue]
  sClCddSigIn_AD_s32ModFlapFroRIFbRawValue/1 -> [sClCddSigIn_AD_s32ModFlapFroRIFbRawValue]
  sClCddSigIn_AD_s32TempFlapFroRIFbRawValue/1 -> [sClCddSigIn_AD_s32TempFlapFroRIFbRawValue]
  sClCddSigIn_AD_s32TempFlapFroLiFbRawValue/1 -> [sClCddSigIn_AD_s32TempFlapFroLiFbRawValue]
  sClCddSigIn_AD_s32RecFlapFbRawValue/1 -> [sClCddSigIn_AD_s32RecFlapFbRawValue]
  sClCddSigIn_AD_s32FroInCarRawValue/1 -> [sClCddSigIn_AD_s32FroInCarRawValue]
  sClCddSigIn_AD_s32HexRawValue/1 -> [sClCddSigIn_AD_s32HexRawValue]
  sClCddSigIn_AD_s32EvapRawValue/1 -> [sClCddSigIn_AD_s32EvapRawValue]
  sClCddSigIn_AD_s32BattRawValue/1 -> [sClCddSigIn_AD_s32BattRawValue]
  [sClCddSigIn_AD_s32RecFlapFbRawValue] -> 319_AVG5/1(sigin)
  311_AVG8/1(sigAvg) -> [sClCddSigProcess_AD_s32ModFlapFroRIFbFilterValue]
  315_AVG10/1(sigAvg) -> [sClCddSigProcess_AD_s32BlowPositivePinFilterValue]
  [sClCddSigIn_AD_s32AqsPinRawValue] -> 312_AVG9/1(sigin)
  312_AVG9/1(sigAvg) -> [sClCddSigProcess_AD_s32AqsPinFilterValue]
  3110_AVG6/1(sigAvg) -> [sClCddSigProcess_AD_s32TempFlapFroLiFbFilterValue]
  [sClCddSigIn_AD_s32ModFlapFroRIFbRawValue] -> 311_AVG8/1(sigin)
  [sClCddSigIn_AD_s32BlowNegativePinRawValue] -> 316_AVG2/1(sigin)
  [sClCddSigIn_AD_s32EvapRawValue] -> 314_AVG1/1(sigin)
  [sClCddSigIn_AD_s32BattRawValue] -> 313_AVG/1(sigin)
  313_AVG/1(sigAvg) -> [sClCddSigProcess_AD_s32BattFilterValue]
  314_AVG1/1(sigAvg) -> [sClCddSigProcess_AD_s32EvapFilterValue]
  319_AVG5/1(sigAvg) -> [sClCddSigProcess_AD_s32RecFlapFbFilterValue]
  [sClCddSigIn_AD_s32FroInCarRawValue] -> 318_AVG4/1(sigin)
  318_AVG4/1(sigAvg) -> [sClCddSigProcess_AD_s32FroInCarFilterValue]
  316_AVG2/1(sigAvg) -> [sClCddSigProcess_AD_s32BlowNegativePinFilterValue]
  [sClCddSigIn_AD_s32TempFlapFroRIFbRawValue] -> 3111_AVG7/1(sigin)
  [sClCddSigIn_AD_s32BlowPositivePinRawValue] -> 315_AVG10/1(sigin)
  [sClCddSigIn_AD_s32HexRawValue] -> 317_AVG3/1(sigin)
  317_AVG3/1(sigAvg) -> [sClCddSigProcess_AD_s32HexFilterValue]
  [sClCddSigIn_AD_s32TempFlapFroLiFbRawValue] -> 3110_AVG6/1(sigin)
  3111_AVG7/1(sigAvg) -> [sClCddSigProcess_AD_s32TempFlapFroRiFbFilterValue]

== system SigProcess/SigProcessSub/Stp6_createPortGotoUpdate/CLHB02001_AdFilter/AVG ==
  note: <模型信息: AVG>
      |
      |
      | 【输入端口】
      | sigin
      |
      | 【输出端口】
      | sigAvg
      |
      | 【标定量】
      | cClCddAdc_D_u8FilterType=
      | cClCddAdc_D_u8RawValueNum=
      |
      | 创建时间: 2025-06-10 10:22:07
  sigin : Inport
  Compare To Constant : simulink/Logic and Bit Operations/Compare To Constant  relop===  const=0  OutDataTypeStr=boolean
  Constant : Constant  Value=cClCddAdc_D_u8FilterType  OutDataTypeStr=uint8
  Constant1 : Constant  Value=cClCddAdc_D_u8RawValueNum  OutDataTypeStr=uint8
  Constant2 : Constant  Commented=on  Value=cTmAfCtrl_Te_s32ShttrPosnColdOnHp
  Counter Limited : simulink/Sources/Counter Limited  uplimit=cClCddAdc_D_u8RawValueNum-1  tsamp=-1
  Data Store Memory : DataStoreMemory  DataStoreName=BattRaw  ReadBeforeWriteMsg=warning  WriteAfterWriteMsg=warning  WriteAfterReadMsg=warning  ShowAdditionalParam=off  OutDataTypeStr=single  Dimensions=[1 20]
      settings: CopyFcn=set_param(gcbh,'ShowName','off');
  Data Store Read : DataStoreRead  DataStoreName=BattRaw  IndexOptions=Index vector (dialog)  Indices=1  OutputSizes=1
  Data Store Write : DataStoreWrite  DataStoreName=BattRaw  DataStoreElements=BattRaw  EnableIndexing=on  IndexMode=Zero-based  IndexOptions=Index vector (port)  Indices=1  OutputSizes=1
  Data Type Conversion : DataTypeConversion  OutDataTypeStr=single  SaturateOnIntegerOverflow=off  RndMeth=Floor
  Gain1 : Gain  Gain=1/cClCddAdc_D_u8RawValueNum
  MATLAB Function : MATLAB Function  TreatAsAtomicUnit=on
  Multiport Switch : MultiPortSwitch  DataPortOrder=Zero-based contiguous  Inputs=5  DataPortForDefault=Additional data port  zeroidx=on  OutDataTypeStr=single  SaturateOnIntegerOverflow=off  InputSameDT=off
  Scope : Scope
  Sum of Elements1 : Sum  Inputs=+
  Switch : Switch  Criteria=u2 ~= 0  SaturateOnIntegerOverflow=off  InputSameDT=off
  Terminator : Terminator  Commented=on
  Unit Delay : UnitDelay  SampleTime=-1  HasFrameUpgradeWarning=on
  sigAvg : Outport  OutDataTypeStr=single
  wires:
  Data Store Read/1 -> MATLAB Function/1(u), Sum of Elements1/1
  Sum of Elements1/1 -> Gain1/1
  Compare To Constant/1 -> Switch/2
  Switch/1 -> [sigAvgSimple], Unit Delay/1
  Gain1/1 -> Switch/1, [sigAvgQuick]
  Counter Limited/1 -> Compare To Constant/1, Data Store Write/2
  Data Type Conversion/1 -> [siginSingle], Data Store Write/1, Scope/1
  MATLAB Function/2(withoutEdge) -> [sigAvgSortWithoutEdge]
  Unit Delay/1 -> Switch/3
  MATLAB Function/1(mid) -> [sigAvgSortedMid]
  sigin/1 -> [sigin]
  [sigin] -> Data Type Conversion/1
  [sigin] -> Multiport Switch/7
  Constant/1 -> Multiport Switch/1
  [sigAvgSortedMid] -> Multiport Switch/3
  [sigAvgSortWithoutEdge] -> Multiport Switch/4
  [sigAvgSimple] -> Multiport Switch/5
  [sigAvgQuick] -> Multiport Switch/6
  [siginSingle] -> Multiport Switch/2
  [sigAvg] -> sigAvg/1
  Constant1/1 -> MATLAB Function/2(num)
  Multiport Switch/1 -> [sigAvg]
  Constant2/1 -> Terminator/1

== system SigProcess/SigProcessSub/Stp6_createPortGotoUpdate/CLHB02001_AdFilter/AVG1 ==
  sigin : Inport
  Compare To Constant : simulink/Logic and Bit Operations/Compare To Constant  relop===  const=0  OutDataTypeStr=boolean
  Constant : Constant  Value=cClCddAdc_D_u8FilterType  OutDataTypeStr=uint8
  Constant1 : Constant  Value=cClCddAdc_D_u8RawValueNum  OutDataTypeStr=uint8
  Counter Limited : simulink/Sources/Counter Limited  uplimit=cClCddAdc_D_u8RawValueNum-1  tsamp=-1
  Data Store Memory : DataStoreMemory  DataStoreName=EvapRaw  ReadBeforeWriteMsg=warning  WriteAfterWriteMsg=warning  WriteAfterReadMsg=warning  ShowAdditionalParam=off  OutDataTypeStr=single  Dimensions=[1 20]
      settings: CopyFcn=set_param(gcbh,'ShowName','off');
  Data Store Read : DataStoreRead  DataStoreName=EvapRaw  IndexOptions=Index vector (dialog)  Indices=1  OutputSizes=1
  Data Store Write : DataStoreWrite  DataStoreName=EvapRaw  DataStoreElements=EvapRaw  EnableIndexing=on  IndexMode=Zero-based  IndexOptions=Index vector (port)  Indices=1  OutputSizes=1
  Data Type Conversion : DataTypeConversion  OutDataTypeStr=single  SaturateOnIntegerOverflow=off  RndMeth=Floor
  Gain1 : Gain  Gain=1/cClCddAdc_D_u8RawValueNum
  MATLAB Function : MATLAB Function  TreatAsAtomicUnit=on
  Multiport Switch : MultiPortSwitch  DataPortOrder=Zero-based contiguous  Inputs=5  DataPortForDefault=Additional data port  zeroidx=on  OutDataTypeStr=single  SaturateOnIntegerOverflow=off  InputSameDT=off
  Scope : Scope
  Sum of Elements1 : Sum  Inputs=+
  Switch : Switch  Criteria=u2 ~= 0  SaturateOnIntegerOverflow=off  InputSameDT=off
  Unit Delay : UnitDelay  SampleTime=-1  HasFrameUpgradeWarning=on
  sigAvg : Outport  OutDataTypeStr=single
  wires:
  Constant1/1 -> MATLAB Function/2(num)
  [sigAvg] -> sigAvg/1
  Multiport Switch/1 -> [sigAvg]
  [siginSingle] -> Multiport Switch/2
  [sigAvgQuick] -> Multiport Switch/6
  [sigAvgSimple] -> Multiport Switch/5
  [sigAvgSortWithoutEdge] -> Multiport Switch/4
  [sigAvgSortedMid] -> Multiport Switch/3
  Constant/1 -> Multiport Switch/1
  [sigin] -> Multiport Switch/7
  [sigin] -> Data Type Conversion/1
  sigin/1 -> [sigin]
  MATLAB Function/1(mid) -> [sigAvgSortedMid]
  Unit Delay/1 -> Switch/3
  MATLAB Function/2(withoutEdge) -> [sigAvgSortWithoutEdge]
  Data Type Conversion/1 -> Scope/1, Data Store Write/1, [siginSingle]
  Counter Limited/1 -> Data Store Write/2, Compare To Constant/1
  Gain1/1 -> [sigAvgQuick], Switch/1
  Switch/1 -> Unit Delay/1, [sigAvgSimple]
  Compare To Constant/1 -> Switch/2
  Sum of Elements1/1 -> Gain1/1
  Data Store Read/1 -> Sum of Elements1/1, MATLAB Function/1(u)

== system SigProcess/SigProcessSub/Stp6_createPortGotoUpdate/CLHB02001_AdFilter/AVG10 ==
  sigin : Inport
  Compare To Constant : simulink/Logic and Bit Operations/Compare To Constant  relop===  const=0  OutDataTypeStr=boolean
  Constant : Constant  Value=cClCddAdc_D_u8FilterType  OutDataTypeStr=uint8
  Constant1 : Constant  Value=cClCddAdc_D_u8RawValueNum  OutDataTypeStr=uint8
  Counter Limited : simulink/Sources/Counter Limited  uplimit=cClCddAdc_D_u8RawValueNum-1  tsamp=-1
  Data Store Memory : DataStoreMemory  DataStoreName=BlowPositivePinRaw  ReadBeforeWriteMsg=warning  WriteAfterWriteMsg=warning  WriteAfterReadMsg=warning  ShowAdditionalParam=off  OutDataTypeStr=single  Dimensions=[1 20]
      settings: CopyFcn=set_param(gcbh,'ShowName','off');
  Data Store Read : DataStoreRead  DataStoreName=BlowPositivePinRaw  IndexOptions=Index vector (dialog)  Indices=1  OutputSizes=1
  Data Store Write : DataStoreWrite  DataStoreName=BlowPositivePinRaw  DataStoreElements=BlowPositivePinRaw  EnableIndexing=on  IndexMode=Zero-based  IndexOptions=Index vector (port)  Indices=1  OutputSizes=1
  Data Type Conversion : DataTypeConversion  OutDataTypeStr=single  SaturateOnIntegerOverflow=off  RndMeth=Floor
  Gain1 : Gain  Gain=1/cClCddAdc_D_u8RawValueNum
  MATLAB Function : MATLAB Function  TreatAsAtomicUnit=on
  Multiport Switch : MultiPortSwitch  DataPortOrder=Zero-based contiguous  Inputs=5  DataPortForDefault=Additional data port  zeroidx=on  OutDataTypeStr=single  SaturateOnIntegerOverflow=off  InputSameDT=off
  Scope : Scope
  Sum of Elements1 : Sum  Inputs=+
  Switch : Switch  Criteria=u2 ~= 0  SaturateOnIntegerOverflow=off  InputSameDT=off
  Unit Delay : UnitDelay  SampleTime=-1  HasFrameUpgradeWarning=on
  sigAvg : Outport  OutDataTypeStr=single
  wires:
  Data Store Read/1 -> MATLAB Function/1(u), Sum of Elements1/1
  Sum of Elements1/1 -> Gain1/1
  Compare To Constant/1 -> Switch/2
  Switch/1 -> [sigAvgSimple], Unit Delay/1
  Gain1/1 -> Switch/1, [sigAvgQuick]
  Counter Limited/1 -> Compare To Constant/1, Data Store Write/2
  Data Type Conversion/1 -> [siginSingle], Data Store Write/1, Scope/1
  MATLAB Function/2(withoutEdge) -> [sigAvgSortWithoutEdge]
  Unit Delay/1 -> Switch/3
  MATLAB Function/1(mid) -> [sigAvgSortedMid]
  sigin/1 -> [sigin]
  [sigin] -> Data Type Conversion/1
  [sigin] -> Multiport Switch/7
  Constant/1 -> Multiport Switch/1
  [sigAvgSortedMid] -> Multiport Switch/3
  [sigAvgSortWithoutEdge] -> Multiport Switch/4
  [sigAvgSimple] -> Multiport Switch/5
  [sigAvgQuick] -> Multiport Switch/6
  [siginSingle] -> Multiport Switch/2
  Multiport Switch/1 -> [sigAvg]
  [sigAvg] -> sigAvg/1
  Constant1/1 -> MATLAB Function/2(num)

== system SigProcess/SigProcessSub/Stp6_createPortGotoUpdate/CLHB02001_AdFilter/AVG2 ==
  sigin : Inport
  Compare To Constant : simulink/Logic and Bit Operations/Compare To Constant  relop===  const=0  OutDataTypeStr=boolean
  Constant : Constant  Value=cClCddAdc_D_u8FilterType  OutDataTypeStr=uint8
  Constant1 : Constant  Value=cClCddAdc_D_u8RawValueNum  OutDataTypeStr=uint8
  Counter Limited : simulink/Sources/Counter Limited  uplimit=cClCddAdc_D_u8RawValueNum-1  tsamp=-1
  Data Store Memory : DataStoreMemory  DataStoreName=BlowNegativePinRaw  ReadBeforeWriteMsg=warning  WriteAfterWriteMsg=warning  WriteAfterReadMsg=warning  ShowAdditionalParam=off  OutDataTypeStr=single  Dimensions=[1 20]
      settings: CopyFcn=set_param(gcbh,'ShowName','off');
  Data Store Read : DataStoreRead  DataStoreName=BlowNegativePinRaw  IndexOptions=Index vector (dialog)  Indices=1  OutputSizes=1
  Data Store Write : DataStoreWrite  DataStoreName=BlowNegativePinRaw  DataStoreElements=BlowNegativePinRaw  EnableIndexing=on  IndexMode=Zero-based  IndexOptions=Index vector (port)  Indices=1  OutputSizes=1
  Data Type Conversion : DataTypeConversion  OutDataTypeStr=single  SaturateOnIntegerOverflow=off  RndMeth=Floor
  Gain1 : Gain  Gain=1/cClCddAdc_D_u8RawValueNum
  MATLAB Function : MATLAB Function  TreatAsAtomicUnit=on
  Multiport Switch : MultiPortSwitch  DataPortOrder=Zero-based contiguous  Inputs=5  DataPortForDefault=Additional data port  zeroidx=on  OutDataTypeStr=single  SaturateOnIntegerOverflow=off  InputSameDT=off
  Scope : Scope
  Sum of Elements1 : Sum  Inputs=+
  Switch : Switch  Criteria=u2 ~= 0  SaturateOnIntegerOverflow=off  InputSameDT=off
  Unit Delay : UnitDelay  SampleTime=-1  HasFrameUpgradeWarning=on
  sigAvg : Outport  OutDataTypeStr=single
  wires:
  Data Store Read/1 -> MATLAB Function/1(u), Sum of Elements1/1
  Sum of Elements1/1 -> Gain1/1
  Compare To Constant/1 -> Switch/2
  Switch/1 -> [sigAvgSimple], Unit Delay/1
  Gain1/1 -> Switch/1, [sigAvgQuick]
  Counter Limited/1 -> Compare To Constant/1, Data Store Write/2
  Data Type Conversion/1 -> [siginSingle], Data Store Write/1, Scope/1
  MATLAB Function/2(withoutEdge) -> [sigAvgSortWithoutEdge]
  Unit Delay/1 -> Switch/3
  MATLAB Function/1(mid) -> [sigAvgSortedMid]
  sigin/1 -> [sigin]
  [sigin] -> Data Type Conversion/1
  [sigin] -> Multiport Switch/7
  Constant/1 -> Multiport Switch/1
  [sigAvgSortedMid] -> Multiport Switch/3
  [sigAvgSortWithoutEdge] -> Multiport Switch/4
  [sigAvgSimple] -> Multiport Switch/5
  [sigAvgQuick] -> Multiport Switch/6
  [siginSingle] -> Multiport Switch/2
  Multiport Switch/1 -> [sigAvg]
  [sigAvg] -> sigAvg/1
  Constant1/1 -> MATLAB Function/2(num)

== system SigProcess/SigProcessSub/Stp6_createPortGotoUpdate/CLHB02001_AdFilter/AVG3 ==
  sigin : Inport
  Compare To Constant : simulink/Logic and Bit Operations/Compare To Constant  relop===  const=0  OutDataTypeStr=boolean
  Constant : Constant  Value=cClCddAdc_D_u8FilterType  OutDataTypeStr=uint8
  Constant1 : Constant  Value=cClCddAdc_D_u8RawValueNum  OutDataTypeStr=uint8
  Counter Limited : simulink/Sources/Counter Limited  uplimit=cClCddAdc_D_u8RawValueNum-1  tsamp=-1
  Data Store Memory : DataStoreMemory  DataStoreName=HexRaw  ReadBeforeWriteMsg=warning  WriteAfterWriteMsg=warning  WriteAfterReadMsg=warning  ShowAdditionalParam=off  OutDataTypeStr=single  Dimensions=[1 20]
      settings: CopyFcn=set_param(gcbh,'ShowName','off');
  Data Store Read : DataStoreRead  DataStoreName=HexRaw  IndexOptions=Index vector (dialog)  Indices=1  OutputSizes=1
  Data Store Write : DataStoreWrite  DataStoreName=HexRaw  DataStoreElements=HexRaw  EnableIndexing=on  IndexMode=Zero-based  IndexOptions=Index vector (port)  Indices=1  OutputSizes=1
  Data Type Conversion : DataTypeConversion  OutDataTypeStr=single  SaturateOnIntegerOverflow=off  RndMeth=Floor
  Gain1 : Gain  Gain=1/cClCddAdc_D_u8RawValueNum
  MATLAB Function : MATLAB Function  TreatAsAtomicUnit=on
  Multiport Switch : MultiPortSwitch  DataPortOrder=Zero-based contiguous  Inputs=5  DataPortForDefault=Additional data port  zeroidx=on  OutDataTypeStr=single  SaturateOnIntegerOverflow=off  InputSameDT=off
  Scope : Scope
  Sum of Elements1 : Sum  Inputs=+
  Switch : Switch  Criteria=u2 ~= 0  SaturateOnIntegerOverflow=off  InputSameDT=off
  Unit Delay : UnitDelay  SampleTime=-1  HasFrameUpgradeWarning=on
  sigAvg : Outport  OutDataTypeStr=single
  wires:
  Constant1/1 -> MATLAB Function/2(num)
  [sigAvg] -> sigAvg/1
  Multiport Switch/1 -> [sigAvg]
  [siginSingle] -> Multiport Switch/2
  [sigAvgQuick] -> Multiport Switch/6
  [sigAvgSimple] -> Multiport Switch/5
  [sigAvgSortWithoutEdge] -> Multiport Switch/4
  [sigAvgSortedMid] -> Multiport Switch/3
  Constant/1 -> Multiport Switch/1
  [sigin] -> Multiport Switch/7
  [sigin] -> Data Type Conversion/1
  sigin/1 -> [sigin]
  MATLAB Function/1(mid) -> [sigAvgSortedMid]
  Unit Delay/1 -> Switch/3
  MATLAB Function/2(withoutEdge) -> [sigAvgSortWithoutEdge]
  Data Type Conversion/1 -> Scope/1, Data Store Write/1, [siginSingle]
  Counter Limited/1 -> Data Store Write/2, Compare To Constant/1
  Gain1/1 -> [sigAvgQuick], Switch/1
  Switch/1 -> Unit Delay/1, [sigAvgSimple]
  Compare To Constant/1 -> Switch/2
  Sum of Elements1/1 -> Gain1/1
  Data Store Read/1 -> Sum of Elements1/1, MATLAB Function/1(u)

== system SigProcess/SigProcessSub/Stp6_createPortGotoUpdate/CLHB02001_AdFilter/AVG4 ==
  sigin : Inport
  Compare To Constant : simulink/Logic and Bit Operations/Compare To Constant  relop===  const=0  OutDataTypeStr=boolean
  Constant : Constant  Value=cClCddAdc_D_u8FilterType  OutDataTypeStr=uint8
  Constant1 : Constant  Value=cClCddAdc_D_u8RawValueNum  OutDataTypeStr=uint8
  Counter Limited : simulink/Sources/Counter Limited  uplimit=cClCddAdc_D_u8RawValueNum-1  tsamp=-1
  Data Store Memory : DataStoreMemory  DataStoreName=FroInCarRaw  ReadBeforeWriteMsg=warning  WriteAfterWriteMsg=warning  WriteAfterReadMsg=warning  ShowAdditionalParam=off  OutDataTypeStr=single  Dimensions=[1 20]
      settings: CopyFcn=set_param(gcbh,'ShowName','off');
  Data Store Read : DataStoreRead  DataStoreName=FroInCarRaw  IndexOptions=Index vector (dialog)  Indices=1  OutputSizes=1
  Data Store Write : DataStoreWrite  DataStoreName=FroInCarRaw  DataStoreElements=FroInCarRaw  EnableIndexing=on  IndexMode=Zero-based  IndexOptions=Index vector (port)  Indices=1  OutputSizes=1
  Data Type Conversion : DataTypeConversion  OutDataTypeStr=single  SaturateOnIntegerOverflow=off  RndMeth=Floor
  Gain1 : Gain  Gain=1/cClCddAdc_D_u8RawValueNum
  MATLAB Function : MATLAB Function  TreatAsAtomicUnit=on
  Multiport Switch : MultiPortSwitch  DataPortOrder=Zero-based contiguous  Inputs=5  DataPortForDefault=Additional data port  zeroidx=on  OutDataTypeStr=single  SaturateOnIntegerOverflow=off  InputSameDT=off
  Scope : Scope
  Sum of Elements1 : Sum  Inputs=+
  Switch : Switch  Criteria=u2 ~= 0  SaturateOnIntegerOverflow=off  InputSameDT=off
  Unit Delay : UnitDelay  SampleTime=-1  HasFrameUpgradeWarning=on
  sigAvg : Outport  OutDataTypeStr=single
  wires:
  Data Store Read/1 -> MATLAB Function/1(u), Sum of Elements1/1
  Sum of Elements1/1 -> Gain1/1
  Compare To Constant/1 -> Switch/2
  Switch/1 -> [sigAvgSimple], Unit Delay/1
  Gain1/1 -> Switch/1, [sigAvgQuick]
  Counter Limited/1 -> Compare To Constant/1, Data Store Write/2
  Data Type Conversion/1 -> [siginSingle], Data Store Write/1, Scope/1
  MATLAB Function/2(withoutEdge) -> [sigAvgSortWithoutEdge]
  Unit Delay/1 -> Switch/3
  MATLAB Function/1(mid) -> [sigAvgSortedMid]
  sigin/1 -> [sigin]
  [sigin] -> Data Type Conversion/1
  [sigin] -> Multiport Switch/7
  Constant/1 -> Multiport Switch/1
  [sigAvgSortedMid] -> Multiport Switch/3
  [sigAvgSortWithoutEdge] -> Multiport Switch/4
  [sigAvgSimple] -> Multiport Switch/5
  [sigAvgQuick] -> Multiport Switch/6
  [siginSingle] -> Multiport Switch/2
  Multiport Switch/1 -> [sigAvg]
  [sigAvg] -> sigAvg/1
  Constant1/1 -> MATLAB Function/2(num)

== system SigProcess/SigProcessSub/Stp6_createPortGotoUpdate/CLHB02001_AdFilter/AVG5 ==
  sigin : Inport
  Compare To Constant : simulink/Logic and Bit Operations/Compare To Constant  relop===  const=0  OutDataTypeStr=boolean
  Constant : Constant  Value=cClCddAdc_D_u8FilterType  OutDataTypeStr=uint8
  Constant1 : Constant  Value=cClCddAdc_D_u8RawValueNum  OutDataTypeStr=uint8
  Counter Limited : simulink/Sources/Counter Limited  uplimit=cClCddAdc_D_u8RawValueNum-1  tsamp=-1
  Data Store Memory : DataStoreMemory  DataStoreName=RecFlapFbRaw  ReadBeforeWriteMsg=warning  WriteAfterWriteMsg=warning  WriteAfterReadMsg=warning  ShowAdditionalParam=off  OutDataTypeStr=single  Dimensions=[1 20]
      settings: CopyFcn=set_param(gcbh,'ShowName','off');
  Data Store Read : DataStoreRead  DataStoreName=RecFlapFbRaw  IndexOptions=Index vector (dialog)  Indices=1  OutputSizes=1
  Data Store Write : DataStoreWrite  DataStoreName=RecFlapFbRaw  DataStoreElements=RecFlapFbRaw  EnableIndexing=on  IndexMode=Zero-based  IndexOptions=Index vector (port)  Indices=1  OutputSizes=1
  Data Type Conversion : DataTypeConversion  OutDataTypeStr=single  SaturateOnIntegerOverflow=off  RndMeth=Floor
  Gain1 : Gain  Gain=1/cClCddAdc_D_u8RawValueNum
  MATLAB Function : MATLAB Function  TreatAsAtomicUnit=on
  Multiport Switch : MultiPortSwitch  DataPortOrder=Zero-based contiguous  Inputs=5  DataPortForDefault=Additional data port  zeroidx=on  OutDataTypeStr=single  SaturateOnIntegerOverflow=off  InputSameDT=off
  Scope : Scope
  Sum of Elements1 : Sum  Inputs=+
  Switch : Switch  Criteria=u2 ~= 0  SaturateOnIntegerOverflow=off  InputSameDT=off
  Unit Delay : UnitDelay  SampleTime=-1  HasFrameUpgradeWarning=on
  sigAvg : Outport  OutDataTypeStr=single
  wires:
  Constant1/1 -> MATLAB Function/2(num)
  [sigAvg] -> sigAvg/1
  Multiport Switch/1 -> [sigAvg]
  [siginSingle] -> Multiport Switch/2
  [sigAvgQuick] -> Multiport Switch/6
  [sigAvgSimple] -> Multiport Switch/5
  [sigAvgSortWithoutEdge] -> Multiport Switch/4
  [sigAvgSortedMid] -> Multiport Switch/3
  Constant/1 -> Multiport Switch/1
  [sigin] -> Multiport Switch/7
  [sigin] -> Data Type Conversion/1
  sigin/1 -> [sigin]
  MATLAB Function/1(mid) -> [sigAvgSortedMid]
  Unit Delay/1 -> Switch/3
  MATLAB Function/2(withoutEdge) -> [sigAvgSortWithoutEdge]
  Data Type Conversion/1 -> Scope/1, Data Store Write/1, [siginSingle]
  Counter Limited/1 -> Data Store Write/2, Compare To Constant/1
  Gain1/1 -> [sigAvgQuick], Switch/1
  Switch/1 -> Unit Delay/1, [sigAvgSimple]
  Compare To Constant/1 -> Switch/2
  Sum of Elements1/1 -> Gain1/1
  Data Store Read/1 -> Sum of Elements1/1, MATLAB Function/1(u)
